simulink model "PT_Grip"  (R2016b)
settings: configuration reference "CodeGenConfigSet" (kept outside this file)
values from neighbouring files (symbols this model uses):
  NOT_AVL = uint8(0)    [init_PT_Grip.m]    (also in init_PT_Grip_SIL.m)
  PT_GripCfg_CW = Calibration.Parameter    [init_PT_Grip.m]    (also in init_PT_Grip_SIL.m = Simulink.Parameter)
  PT_rClthSlip_C = Calibration.Parameter    [init_PT_Grip.m]    (also in init_PT_Grip_SIL.m = Simulink.Parameter)
  PT_rClthSlipDeb_C = Calibration.Parameter    [init_PT_Grip.m]    (also in init_PT_Grip_SIL.m = Simulink.Parameter)
  PT_rGrip_C = Calibration.Parameter    [init_PT_Grip.m]    (also in init_PT_Grip_SIL.m = Simulink.Parameter)
  PT_rGripDfl_C = Calibration.Parameter    [init_PT_Grip.m]    (also in init_PT_Grip_SIL.m = Simulink.Parameter)
  PT_rNoGrip_C = Calibration.Parameter    [init_PT_Grip.m]    (also in init_PT_Grip_SIL.m = Simulink.Parameter)
  PT_tiDebClthStSlip_C = Calibration.Parameter    [init_PT_Grip.m]    (also in init_PT_Grip_SIL.m = Simulink.Parameter)
  PT_vMinGrip_C = Calibration.Parameter    [init_PT_Grip.m]    (also in init_PT_Grip_SIL.m = Simulink.Parameter)
  TRA_INTERLOCK_SY = uint8(1)    [init_PT_Grip.m]    (also in init_PT_Grip_SIL.m)
  TRA_MT_SY = uint8(1)    [init_PT_Grip.m]    (also in init_PT_Grip_SIL.m)
undefined symbols (not defined in the file or in its folder): PT_Grip_DT, PT_TraType_State_conv
libraries: simulink x5, CXLib x1
settings Model: Creator=Administrator  LastModifiedBy=lenovo
settings ConfigSetRef: SourceLocation=Base Workspace

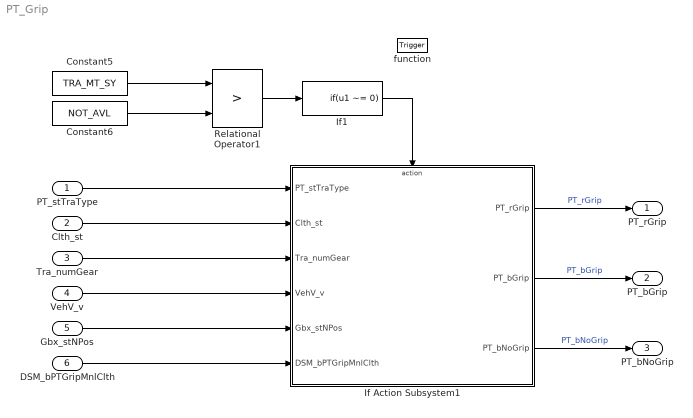
== system PT_Grip ==
  PT_stTraType : Inport  Description=Current transmission type  OutDataTypeStr=Enum: PT_TraType_State_conv
  Clth_st : Inport  Description=Clutch information  Port=2  OutMin=0  OutMax=255  OutDataTypeStr=State_uint8
  Tra_numGear : Inport  Description=Current gear information  Port=3  OutMin=-128  OutMax=127  OutDataTypeStr=Tra_num
  VehV_v : Inport  Tag=km/h  Description=Vehicle speed  Port=4  OutMin=0  OutMax=250  OutDataTypeStr=VehSpeed_km_h
  Gbx_stNPos : Inport  Description=Gearbox neutral position status signal  Port=5  OutMin=0  OutMax=255  OutDataTypeStr=State_uint8
  DSM_bPTGripMnlClth : Inport  Description=Status of FId_PTGripMnlClth  Port=6  OutMin=0  OutMax=1  OutDataTypeStr=boolean
  function : TriggerPort  TriggerType=function-call  VariantControl=Variant
  Constant5 : Constant  RequirementInfo={'other' 'APP_requirements.doc' '@Simulink_requirement_item_25' 'true' '手动开关' '' } %GIDa_1c56857f_248e_4fa6_8b6c_5bec6f457af3  Value=TRA_MT_SY
  Constant6 : Constant  RequirementInfo={'other' 'APP_requirements.doc' '@Simulink_requirement_item_25' 'true' '手动开关' '' } %GIDa_608eb77d_4249_476e_93b7_eeb78d3240d6  Value=NOT_AVL  OutDataTypeStr=Inherit: Inherit via back propagation
  If Action Subsystem1 : Subsystem  TreatAsAtomicUnit=on
  If1 : If  IfExpression=u1 ~= 0  ShowElse=off
  Relational Operator1 : RelationalOperator  Operator=>  OutDataTypeStr=boolean  RndMeth=Simplest  InputSameDT=on
  PT_rGrip : Outport  Description=Analogue value for the grip states  OutMin=-300  OutMax=300  OutDataTypeStr=Prc_Fact100
  PT_bGrip : Outport  Description=Grip is for sure present (the converter lockup clutch / the automated or manual clutch is completely closed and PT_bNoGrip = FALSE)  Port=2  OutMin=0  OutMax=1  OutDataTypeStr=boolean
  PT_bNoGrip : Outport  Description=Grip reliable exclude  Port=3  OutMin=0  OutMax=1  OutDataTypeStr=boolean
  wires:
  If Action Subsystem1/1(PT_rGrip) -> PT_rGrip/1  "PT_rGrip"
  If Action Subsystem1/2(PT_bGrip) -> PT_bGrip/1  "PT_bGrip"
  If Action Subsystem1/3(PT_bNoGrip) -> PT_bNoGrip/1  "PT_bNoGrip"
  If1/1 -> If Action Subsystem1/Action
  Relational Operator1/1 -> If1/1
  Constant5/1 -> Relational Operator1/1
  Constant6/1 -> Relational Operator1/2
  PT_stTraType/1 -> If Action Subsystem1/1(PT_stTraType)
  Clth_st/1 -> If Action Subsystem1/2(Clth_st)
  Tra_numGear/1 -> If Action Subsystem1/3(Tra_numGear)
  VehV_v/1 -> If Action Subsystem1/4(VehV_v)
  Gbx_stNPos/1 -> If Action Subsystem1/5(Gbx_stNPos)
  DSM_bPTGripMnlClth/1 -> If Action Subsystem1/6(DSM_bPTGripMnlClth)

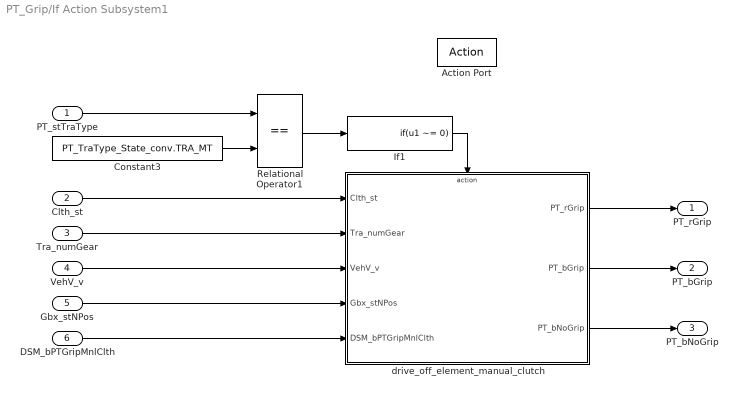
== system PT_Grip/If Action Subsystem1 ==
  PT_stTraType : Inport  Description=Current transmission type  OutDataTypeStr=Enum: PT_TraType_State_conv
  Clth_st : Inport  Description=Clutch information  Port=2  OutMin=0  OutMax=255
  Tra_numGear : Inport  Description=Current gear information  Port=3  OutMin=-128  OutMax=127  OutDataTypeStr=Tra_num
  VehV_v : Inport  Tag=km/h  Description=Vehicle speed  Port=4  OutMin=0  OutMax=250  OutDataTypeStr=VehSpeed_km_h
  Gbx_stNPos : Inport  Description=Gearbox neutral position status signal  Port=5  OutMin=0  OutMax=255
  DSM_bPTGripMnlClth : Inport  Description=Status of FId_PTGripMnlClth  Port=6  OutMin=0  OutMax=1  OutDataTypeStr=boolean
  Action Port : ActionPort  ActionType=then
  Constant3 : Constant  RequirementInfo={} %GIDa_6c0c820b_2e16_4965_99e0_1bdbbd8c4bc0  Value=PT_TraType_State_conv.TRA_MT  OutDataTypeStr=Inherit: Inherit via back propagation
  If1 : If  IfExpression=u1 ~= 0  ShowElse=off
  Relational Operator1 : RelationalOperator  Operator===  OutDataTypeStr=boolean  RndMeth=Simplest  InputSameDT=on
  drive_off_element_manual_clutch : Subsystem  TreatAsAtomicUnit=on  RTWFcnName=MnlClth
      settings: RTWFcnNameOpts=User specified
  PT_rGrip : Outport  Description=Grip is for sure present (the converter lockup clutch / the automated or manual clutch is completely closed and PT_bNoGrip = FALSE)  OutMin=0  OutMax=1
  PT_bGrip : Outport  Description=Grip is for sure present (the converter lockup clutch / the automated or manual clutch is completely closed and PT_bNoGrip = FALSE)  Port=2  OutMin=0  OutMax=1  OutDataTypeStr=boolean
  PT_bNoGrip : Outport  Description=Grip reliable exclude  Port=3  OutMin=0  OutMax=1  OutDataTypeStr=boolean
  wires:
  drive_off_element_manual_clutch/3(PT_bNoGrip) -> PT_bNoGrip/1
  drive_off_element_manual_clutch/1(PT_rGrip) -> PT_rGrip/1
  drive_off_element_manual_clutch/2(PT_bGrip) -> PT_bGrip/1
  Gbx_stNPos/1 -> drive_off_element_manual_clutch/4(Gbx_stNPos)
  VehV_v/1 -> drive_off_element_manual_clutch/3(VehV_v)
  Clth_st/1 -> drive_off_element_manual_clutch/1(Clth_st)
  Tra_numGear/1 -> drive_off_element_manual_clutch/2(Tra_numGear)
  PT_stTraType/1 -> Relational Operator1/1
  If1/1 -> drive_off_element_manual_clutch/Action
  Relational Operator1/1 -> If1/1
  Constant3/1 -> Relational Operator1/2
  DSM_bPTGripMnlClth/1 -> drive_off_element_manual_clutch/5(DSM_bPTGripMnlClth)

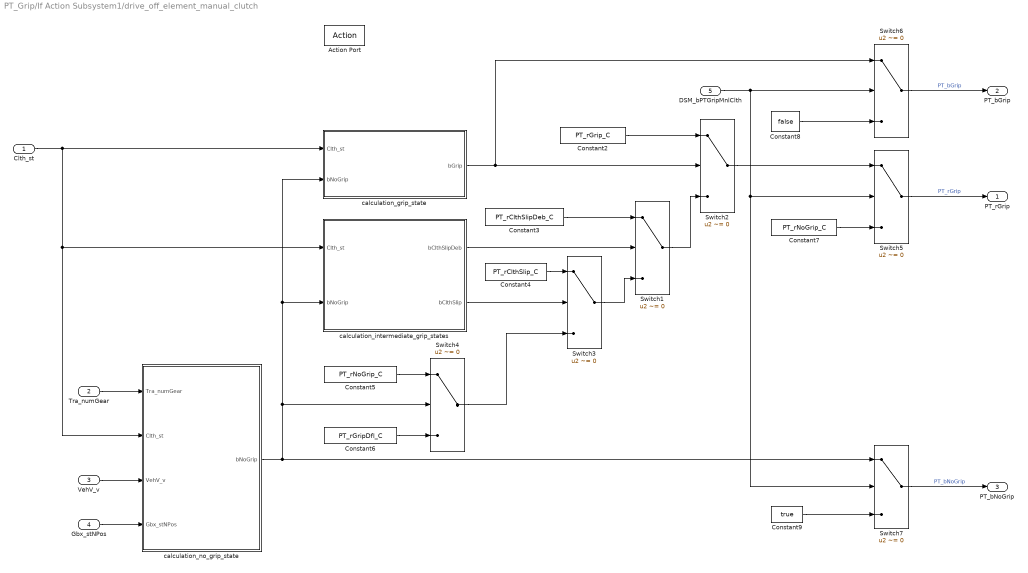
== system PT_Grip/If Action Subsystem1/drive_off_element_manual_clutch ==
  Clth_st : Inport  Description=Clutch information  OutMin=0  OutMax=255
  Tra_numGear : Inport  Description=Current gear information  Port=2  OutMin=-128  OutMax=127  OutDataTypeStr=Tra_num
  VehV_v : Inport  Tag=km/h  Description=Vehicle speed  Port=3  OutMin=0  OutMax=250  OutDataTypeStr=VehSpeed_km_h
  Gbx_stNPos : Inport  Description=Gearbox neutral position status signal  Port=4  OutMin=0  OutMax=255
  DSM_bPTGripMnlClth : Inport  Description=Status of FId_PTGripMnlClth  Port=5  OutMin=0  OutMax=1  OutDataTypeStr=boolean
  Action Port : ActionPort  ActionType=then
  Constant2 : Constant  RequirementInfo={} %GIDa_e4d1f3be_4204_4374_bfd7_d2b75db4c6a2  Value=PT_rGrip_C
  Constant3 : Constant  RequirementInfo={} %GIDa_2d9cf93a_26f0_4bf7_9ad5_70acc211c06d  Value=PT_rClthSlipDeb_C
  Constant4 : Constant  RequirementInfo={} %GIDa_b83e095a_9f93_4737_9f3c_ba346d2b460b  Value=PT_rClthSlip_C
  Constant5 : Constant  RequirementInfo={} %GIDa_5bccbcc5_b243_4463_97da_a7bb4f5e1bf3  Value=PT_rNoGrip_C
  Constant6 : Constant  RequirementInfo={} %GIDa_f11b91fe_8b3f_4321_a0ad_50de5baa2684  Value=PT_rGripDfl_C
  Constant7 : Constant  RequirementInfo={} %GIDa_2c8c07ac_3f65_4183_8322_85c6724d31c9  Value=PT_rNoGrip_C
  Constant8 : Constant  RequirementInfo={} %GIDa_38976eeb_dab7_44a2_a7bf_c05f7b83b63a  Value=false  OutDataTypeStr=boolean
  Constant9 : Constant  RequirementInfo={} %GIDa_eef7394e_e6f2_4d02_95ef_25cd4ea567b8  Value=true  OutDataTypeStr=Inherit: Inherit via back propagation
  Switch{1..7} (7 alike) : Switch  Criteria=u2 ~= 0  InputSameDT=on
  calculation_grip_state : Subsystem
  calculation_intermediate_grip_states : Subsystem
  calculation_no_grip_state : Subsystem
  PT_rGrip : Outport
  PT_bGrip : Outport  Description=Grip is for sure present (the converter lockup clutch / the automated or manual clutch is completely closed and PT_bNoGrip = FALSE)  Port=2
  PT_bNoGrip : Outport  Port=3
  wires:
  Switch7/1 -> PT_bNoGrip/1  "PT_bNoGrip"
  Constant9/1 -> Switch7/3
  Switch6/1 -> PT_bGrip/1  "PT_bGrip"
  Constant8/1 -> Switch6/3
  Switch5/1 -> PT_rGrip/1  "PT_rGrip"
  Constant7/1 -> Switch5/3
  Switch2/1 -> Switch5/1
  Switch4/1 -> Switch3/3
  Constant6/1 -> Switch4/3
  Constant5/1 -> Switch4/1
  calculation_no_grip_state/1(bNoGrip) -> Switch4/2, calculation_intermediate_grip_states/2(bNoGrip), calculation_grip_state/2(bNoGrip), Switch7/1
  Constant4/1 -> Switch3/1
  calculation_intermediate_grip_states/2(bClthSlip) -> Switch3/2
  Switch3/1 -> Switch1/3
  Constant3/1 -> Switch1/1
  Switch1/1 -> Switch2/3
  Constant2/1 -> Switch2/1
  Gbx_stNPos/1 -> calculation_no_grip_state/4(Gbx_stNPos)
  VehV_v/1 -> calculation_no_grip_state/3(VehV_v)
  Tra_numGear/1 -> calculation_no_grip_state/1(Tra_numGear)
  calculation_intermediate_grip_states/1(bClthSlipDeb) -> Switch1/2
  calculation_grip_state/1(bGrip) -> Switch2/2, Switch6/1
  Clth_st/1 -> calculation_grip_state/1(Clth_st), calculation_no_grip_state/2(Clth_st), calculation_intermediate_grip_states/1(Clth_st)
  DSM_bPTGripMnlClth/1 -> Switch7/2, Switch5/2, Switch6/2

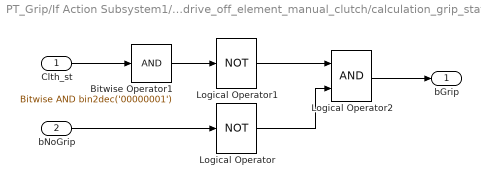
== system PT_Grip/If Action Subsystem1/drive_off_element_manual_clutch/calculation_grip_state ==
  Clth_st : Inport
  bNoGrip : Inport  Port=2
  Bitwise Operator1 : simulink/Logic and Bit Operations/Bitwise Operator  logicop=AND  UseBitMask=on  BitMask=bin2dec('00000001')  BitMaskRealWorld=Stored Integer
  Logical Operator : Logic  Operator=NOT  AllPortsSameDT=off  OutDataTypeStr=boolean
  Logical Operator1 : Logic  Operator=NOT  AllPortsSameDT=off  OutDataTypeStr=boolean
  Logical Operator2 : Logic  OutDataTypeStr=boolean
  bGrip : Outport
  wires:
  Logical Operator/1 -> Logical Operator2/2
  Logical Operator2/1 -> bGrip/1
  Bitwise Operator1/1 -> Logical Operator1/1
  Clth_st/1 -> Bitwise Operator1/1
  Logical Operator1/1 -> Logical Operator2/1
  bNoGrip/1 -> Logical Operator/1

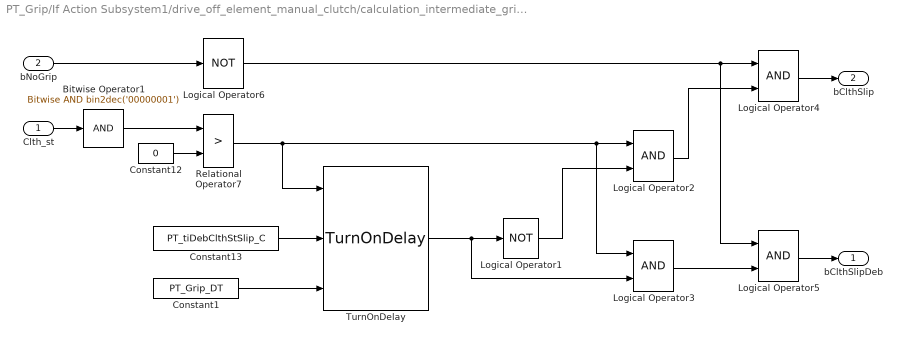
== system PT_Grip/If Action Subsystem1/drive_off_element_manual_clutch/calculation_intermediate_grip_states ==
  Clth_st : Inport
  bNoGrip : Inport  Port=2
  Bitwise Operator1 : simulink/Logic and Bit Operations/Bitwise Operator  logicop=AND  UseBitMask=on  BitMask=bin2dec('00000001')  BitMaskRealWorld=Stored Integer
  Constant1 : Constant  RequirementInfo={} %GIDa_ce3efc46_eb0e_4dfb_89ca_32a0f4b273dc  Value=PT_Grip_DT  OutDataTypeStr=Inherit: Inherit via back propagation
  Constant12 : Constant  RequirementInfo={} %GIDa_563d23b2_ca4c_418b_ab32_28ddda7e13fc  Value=0  OutDataTypeStr=Inherit: Inherit via back propagation
  Constant13 : Constant  RequirementInfo={} %GIDa_f8c7e096_fcef_4fe2_809d_390764efdae1  Value=PT_tiDebClthStSlip_C  SampleTime=-1
  Logical Operator1 : Logic  Operator=NOT  AllPortsSameDT=off  OutDataTypeStr=boolean
  Logical Operator{2..5} (4 alike) : Logic  OutDataTypeStr=boolean
  Logical Operator6 : Logic  Operator=NOT  AllPortsSameDT=off  OutDataTypeStr=boolean
  Relational Operator7 : RelationalOperator  Operator=>  OutDataTypeStr=boolean  RndMeth=Simplest  InputSameDT=on
  TurnOnDelay : CXLib/TurnOnDelay
  bClthSlipDeb : Outport
  bClthSlip : Outport  Port=2
  wires:
  Relational Operator7/1 -> Logical Operator3/1, Logical Operator2/1, TurnOnDelay/1
  Bitwise Operator1/1 -> Relational Operator7/1
  Constant12/1 -> Relational Operator7/2
  Logical Operator1/1 -> Logical Operator2/2
  Logical Operator6/1 -> Logical Operator4/1, Logical Operator5/1
  Logical Operator4/1 -> bClthSlip/1
  Logical Operator3/1 -> Logical Operator5/2
  TurnOnDelay/1 -> Logical Operator1/1, Logical Operator3/2
  Clth_st/1 -> Bitwise Operator1/1
  Logical Operator5/1 -> bClthSlipDeb/1
  Logical Operator2/1 -> Logical Operator4/2
  Constant13/1 -> TurnOnDelay/2
  bNoGrip/1 -> Logical Operator6/1
  Constant1/1 -> TurnOnDelay/3

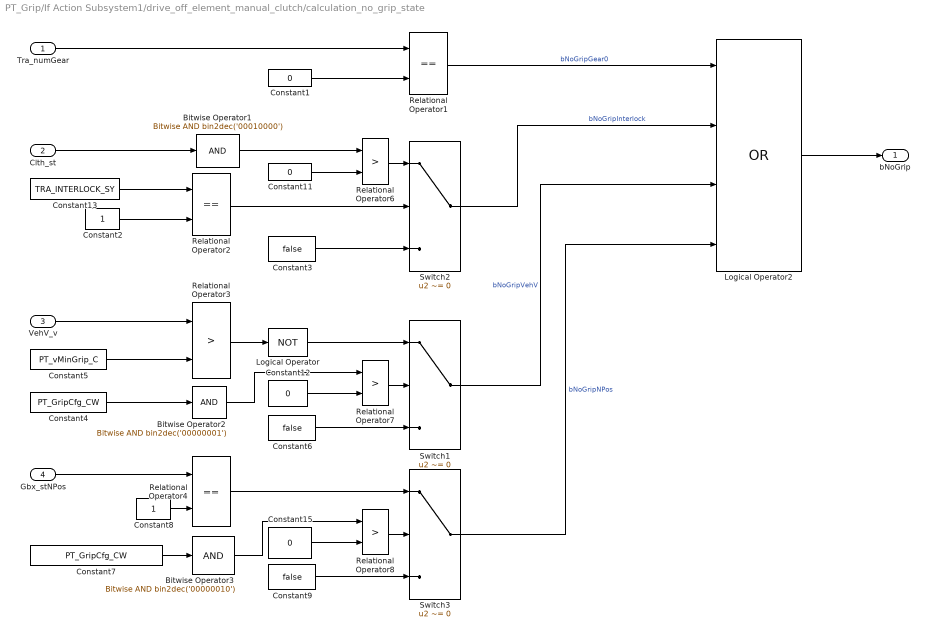
== system PT_Grip/If Action Subsystem1/drive_off_element_manual_clutch/calculation_no_grip_state ==
  Tra_numGear : Inport
  Clth_st : Inport  Port=2  OutDataTypeStr=State_uint8
  VehV_v : Inport  Port=3
  Gbx_stNPos : Inport  Port=4
  Bitwise Operator1 : simulink/Logic and Bit Operations/Bitwise Operator  logicop=AND  UseBitMask=on  BitMask=bin2dec('00010000')  BitMaskRealWorld=Stored Integer
  Bitwise Operator2 : simulink/Logic and Bit Operations/Bitwise Operator  logicop=AND  UseBitMask=on  BitMask=bin2dec('00000001')  BitMaskRealWorld=Stored Integer
  Bitwise Operator3 : simulink/Logic and Bit Operations/Bitwise Operator  logicop=AND  UseBitMask=on  BitMask=bin2dec('00000010')  BitMaskRealWorld=Stored Integer
  Constant1 : Constant  Value=0  OutDataTypeStr=Inherit: Inherit via back propagation
  Constant11 : Constant  RequirementInfo={} %GIDa_63c13eb1_0500_41ed_9653_bfe3b2c7dd16  Value=0  OutDataTypeStr=Inherit: Inherit via back propagation
  Constant12 : Constant  RequirementInfo={} %GIDa_0a5ce1aa_cb9f_4c53_96e3_d3abf6544d8e  Value=0  OutDataTypeStr=Inherit: Inherit via back propagation
  Constant13 : Constant  RequirementInfo={} %GIDa_8264525f_f898_4a58_be78_f858a682d7d9  Value=TRA_INTERLOCK_SY
  Constant15 : Constant  RequirementInfo={} %GIDa_5307a716_51ee_43f4_b106_2cb1b3edfd71  Value=0  OutDataTypeStr=Inherit: Inherit via back propagation
  Constant2 : Constant  OutDataTypeStr=Inherit: Inherit via back propagation
  Constant3 : Constant  RequirementInfo={} %GIDa_6dae603d_6e3b_4822_b545_8b6b02b76ec3  Value=false  OutDataTypeStr=boolean
  Constant4 : Constant  RequirementInfo={} %GIDa_c2583ef7_9862_467c_a96e_309280709d9b  Value=PT_GripCfg_CW
  Constant5 : Constant  RequirementInfo={} %GIDa_456e5813_3b39_47e4_90fb_ddc671dbb6a6  Value=PT_vMinGrip_C
  Constant6 : Constant  Value=false  OutDataTypeStr=boolean
  Constant7 : Constant  RequirementInfo={} %GIDa_6c8d13a9_b659_4097_b290_b3e7ecc3ca47  Value=PT_GripCfg_CW
  Constant8 : Constant  RequirementInfo={} %GIDa_ab604c41_61b7_4601_9cb7_513df1ae8008  OutDataTypeStr=Inherit: Inherit via back propagation
  Constant9 : Constant  Value=false  OutDataTypeStr=boolean
  Logical Operator : Logic  Operator=NOT  AllPortsSameDT=off  OutDataTypeStr=boolean
  Logical Operator2 : Logic  Operator=OR  Inputs=4  OutDataTypeStr=boolean
  Relational Operator1 : RelationalOperator  Operator===  OutDataTypeStr=boolean  RndMeth=Simplest  InputSameDT=on
  Relational Operator2 : RelationalOperator  Operator===  OutDataTypeStr=boolean  RndMeth=Simplest  InputSameDT=on
  Relational Operator{3,6..8} (4 alike) : RelationalOperator  Operator=>  OutDataTypeStr=boolean  RndMeth=Simplest  InputSameDT=on
  Relational Operator4 : RelationalOperator  Operator===  OutDataTypeStr=boolean  RndMeth=Simplest  InputSameDT=on
  Switch1 : Switch  Criteria=u2 ~= 0  InputSameDT=on
  Switch2 : Switch  Criteria=u2 ~= 0  InputSameDT=on
  Switch3 : Switch  Criteria=u2 ~= 0  InputSameDT=on
  bNoGrip : Outport
  wires:
  Bitwise Operator3/1 -> Relational Operator8/1
  Relational Operator8/1 -> Switch3/2
  Constant15/1 -> Relational Operator8/2
  Bitwise Operator2/1 -> Relational Operator7/1
  Relational Operator7/1 -> Switch1/2
  Constant12/1 -> Relational Operator7/2
  Relational Operator6/1 -> Switch2/1
  Constant11/1 -> Relational Operator6/2
  Bitwise Operator1/1 -> Relational Operator6/1
  Constant5/1 -> Relational Operator3/2
  Constant6/1 -> Switch1/3
  Switch3/1 -> Logical Operator2/4  "bNoGripNPos"
  Gbx_stNPos/1 -> Relational Operator4/1
  Constant7/1 -> Bitwise Operator3/1
  Constant9/1 -> Switch3/3
  Constant8/1 -> Relational Operator4/2
  Relational Operator4/1 -> Switch3/1
  Logical Operator2/1 -> bNoGrip/1
  Switch2/1 -> Logical Operator2/2  "bNoGripInterlock"
  Logical Operator/1 -> Switch1/1
  VehV_v/1 -> Relational Operator3/1
  Constant4/1 -> Bitwise Operator2/1
  Constant3/1 -> Switch2/3
  Relational Operator3/1 -> Logical Operator/1
  Constant13/1 -> Relational Operator2/1
  Constant2/1 -> Relational Operator2/2
  Constant1/1 -> Relational Operator1/2
  Tra_numGear/1 -> Relational Operator1/1
  Relational Operator2/1 -> Switch2/2
  Clth_st/1 -> Bitwise Operator1/1
  Switch1/1 -> Logical Operator2/3  "bNoGripVehV"
  Relational Operator1/1 -> Logical Operator2/1  "bNoGripGear0"
